simulink model "penduloInvNoLinealRealimentado"  (Simulink 7.9)
settings: Solver=ode45  StartTime=0.0  StopTime=60  RelTol=1e-3
values from neighbouring files (symbols this model uses):
  K = lqr(A,B,Q,R)    [LQR.m]    (also in bestQ.m = setK_lqr(Q_i); graficosPenduloReal.m = setK_lqr(Q_optimo))
libraries: simulink x5
settings Model: Creator=root  LastModifiedBy=root
settings SFSimCC: SimParseCustomCode=off
settings GRTTargetCC: CombineOutputUpdateFcns=off  GRTInterface=on

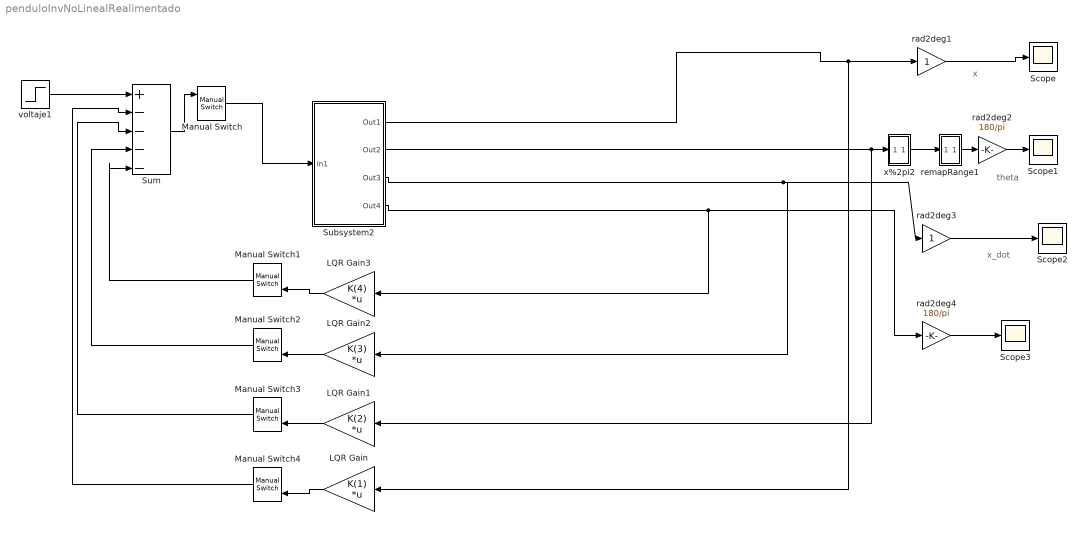
== system penduloInvNoLinealRealimentado ==
  note: x
  note: theta
  note: x_dot
  LQR Gain : Gain  Gain=K(1)  Multiplication=Matrix(K*u)  SaturateOnIntegerOverflow=on  OutDataTypeStr=Inherit: Same as input  ParamDataTypeStr=Inherit: Same as input
  LQR Gain1 : Gain  Gain=K(2)  Multiplication=Matrix(K*u)  SaturateOnIntegerOverflow=on  OutDataTypeStr=Inherit: Same as input  ParamDataTypeStr=Inherit: Same as input
  LQR Gain2 : Gain  Gain=K(3)  Multiplication=Matrix(K*u)  SaturateOnIntegerOverflow=on  OutDataTypeStr=Inherit: Same as input  ParamDataTypeStr=Inherit: Same as input
  LQR Gain3 : Gain  Gain=K(4)  Multiplication=Matrix(K*u)  SaturateOnIntegerOverflow=on  OutDataTypeStr=Inherit: Same as input  ParamDataTypeStr=Inherit: Same as input
  Manual Switch : simulink/Signal Routing/Manual Switch  sw=1  action=0  varsize=off
  Manual Switch{1..4} (4 alike) : simulink/Signal Routing/Manual Switch  sw=0  action=0  varsize=off
  Scope{,1..3} (4 alike) : Scope
      Scope settings: SaveName=ScopeData6
      Scope1 settings: SaveName=ScopeData7
      Scope2 settings: SaveName=ScopeData8
      Scope3 settings: SaveName=ScopeData9
  Subsystem2 : Subsystem
  Sum : Sum  Inputs=|+----
  rad2deg1 : Gain  SaturateOnIntegerOverflow=on  OutDataTypeStr=Inherit: Same as input  ParamDataTypeStr=Inherit: Same as input
  rad2deg2 : Gain  Gain=180/pi  SaturateOnIntegerOverflow=on  OutDataTypeStr=Inherit: Same as input  ParamDataTypeStr=Inherit: Same as input
  rad2deg3 : Gain  SaturateOnIntegerOverflow=on  OutDataTypeStr=Inherit: Same as input  ParamDataTypeStr=Inherit: Same as input
  rad2deg4 : Gain  Gain=180/pi  SaturateOnIntegerOverflow=on  OutDataTypeStr=Inherit: Same as input  ParamDataTypeStr=Inherit: Same as input
  remapRange1 : MATLAB Function  TreatAsAtomicUnit=on
  voltaje1 : Step  Time=0  After=0  SampleTime=0
  x%2pi2 : MATLAB Function  TreatAsAtomicUnit=on
  wires:
  rad2deg4/1 -> Scope3/1
  rad2deg3/1 -> Scope2/1
  Subsystem2/3(Out3) -> LQR Gain2/1, rad2deg3/1
  rad2deg1/1 -> Scope/1
  Subsystem2/1(Out1) -> rad2deg1/1, LQR Gain/1
  Subsystem2/2(Out2) -> LQR Gain1/1, x%2pi2/1(u)
  x%2pi2/1(y) -> remapRange1/1(value)
  LQR Gain3/1 -> Manual Switch1/2
  LQR Gain2/1 -> Manual Switch2/2
  LQR Gain1/1 -> Manual Switch3/2
  LQR Gain/1 -> Manual Switch4/2
  Manual Switch/1 -> Subsystem2/1(In1)
  Subsystem2/4(Out4) -> rad2deg4/1, LQR Gain3/1
  voltaje1/1 -> Sum/1
  Sum/1 -> Manual Switch/1
  Manual Switch1/1 -> Sum/5
  Manual Switch2/1 -> Sum/4
  Manual Switch3/1 -> Sum/3
  Manual Switch4/1 -> Sum/2
  remapRange1/1(y) -> rad2deg2/1
  rad2deg2/1 -> Scope1/1

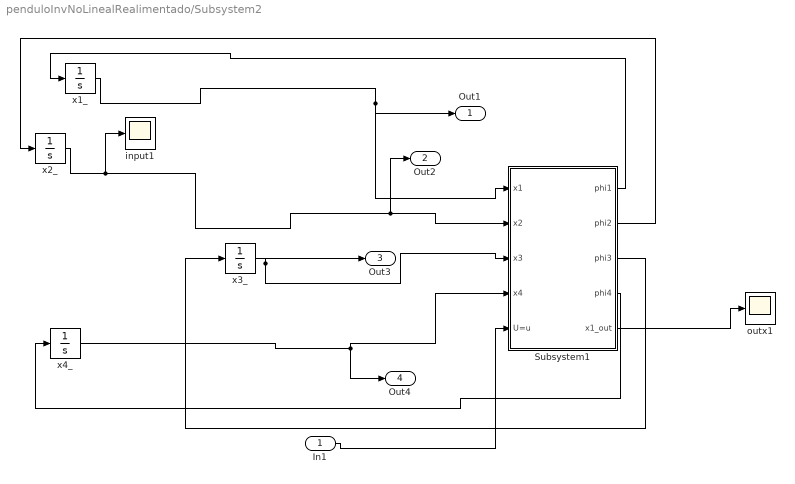
== system penduloInvNoLinealRealimentado/Subsystem2 ==
  In1 : Inport
  Subsystem1 : Subsystem
  input1 : Scope
      settings: SaveName=ScopeData5
  outx1 : Scope
  x1_ : Integrator  LimitOutput=on  UpperSaturationLimit=50  LowerSaturationLimit=-50
  x2_ : Integrator  InitialCondition=170*pi/180  UpperSaturationLimit=2*pi  LowerSaturationLimit=0
  x3_ : Integrator  LimitOutput=on  UpperSaturationLimit=0.5  LowerSaturationLimit=-0.5
  x4_ : Integrator  LimitOutput=on  UpperSaturationLimit=0.5  LowerSaturationLimit=-0.5
  Out1 : Outport
  Out2 : Outport  Port=2
  Out3 : Outport  Port=3
  Out4 : Outport  Port=4
  wires:
  x1_/1 -> Out1/1, Subsystem1/1(x1)
  Subsystem1/1(phi1) -> x1_/1
  Subsystem1/2(phi2) -> x2_/1
  Subsystem1/3(phi3) -> x3_/1
  Subsystem1/4(phi4) -> x4_/1
  x4_/1 -> Out4/1, Subsystem1/4(x4)
  x2_/1 -> input1/1, Out2/1, Subsystem1/2(x2)
  Subsystem1/5(x1_out) -> outx1/1
  In1/1 -> Subsystem1/5(U=u)
  x3_/1 -> Out3/1, Subsystem1/3(x3)

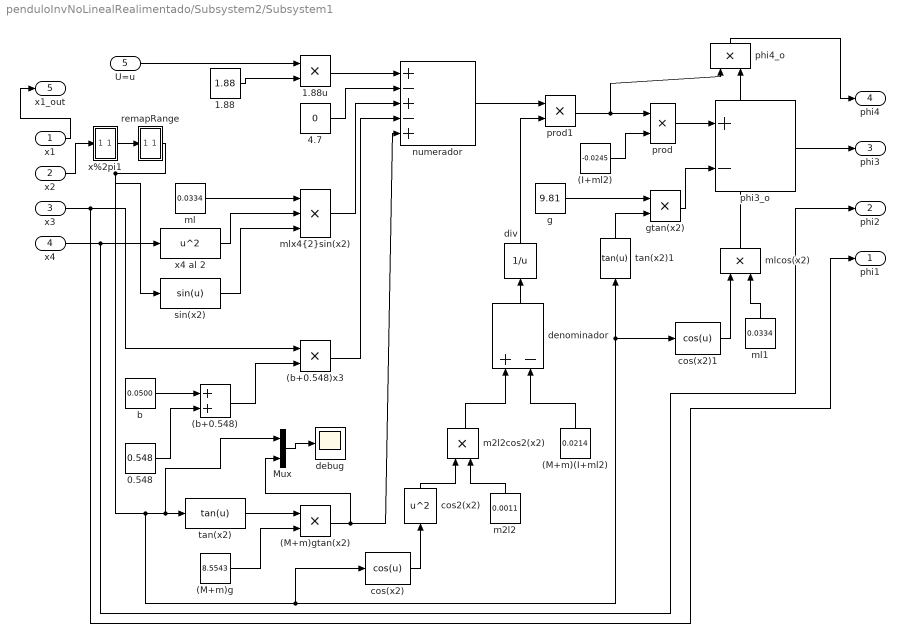
== system penduloInvNoLinealRealimentado/Subsystem2/Subsystem1 ==
  x1 : Inport
  x2 : Inport  Port=2
  x3 : Inport  Port=3
  x4 : Inport  Port=4
  U=u : Inport  Port=5
  (I+ml2) : Constant  Value=-0.0245
  (M+m)(I+ml2) : Constant  Value=0.0214
  (M+m)g : Constant  Value=8.5543
  (M+m)gtan(x2) : Product  RndMeth=Zero
  (b+0.548) : Sum
  (b+0.548)x3 : Product  RndMeth=Zero
  0.548 : Constant  Value=0.548
  1.88 : Constant  Value=1.88
  1.88u : Product  RndMeth=Zero
  4.7 : Constant  Value=0
  Mux : Mux  Inputs=2
  b : Constant  Value=0.0500
  cos(x2) : Fcn  Expr=cos(u)  SampleTime=0.1
  cos(x2)1 : Fcn  Expr=cos(u)  SampleTime=0.1
  cos2(x2) : Fcn  Expr=u^2  SampleTime=0.1
  debug : Scope
      settings: SaveName=debug
  denominador : Sum  Inputs=+-
  div : Fcn  Expr=1/u  SampleTime=0.1
  g : Constant  Value=9.81
  gtan(x2) : Product  RndMeth=Zero
  m2l2 : Constant  Value=0.0011
  m2l2cos2(x2) : Product  RndMeth=Zero
  ml : Constant  Value=0.0334
  ml1 : Constant  Value=0.0334
  mlcos(x2) : Product  RndMeth=Zero
  "mlx4{2}sin(x2)" : Product  Inputs=3  RndMeth=Zero
  numerador : Sum  Inputs=+-+-+
  phi3_o : Sum  Inputs=+-
  phi4_o : Product  RndMeth=Zero
  prod : Product  RndMeth=Zero
  prod1 : Product  RndMeth=Zero
  remapRange : MATLAB Function  TreatAsAtomicUnit=on
  sin(x2) : Fcn  Expr=sin(u)  SampleTime=0.1
  tan(x2) : Fcn  Expr=tan(u)  SampleTime=0.1
  tan(x2)1 : Fcn  Expr=tan(u)  SampleTime=0.1
  x%2pi1 : MATLAB Function  TreatAsAtomicUnit=on
  x4 al 2 : Fcn  Expr=u^2  SampleTime=0.1
  phi1 : Outport
  phi2 : Outport  Port=2
  phi3 : Outport  Port=3
  phi4 : Outport  Port=4
  x1_out : Outport  Port=5
  wires:
  1.88/1 -> 1.88u/2
  U=u/1 -> 1.88u/1
  1.88u/1 -> numerador/1
  4.7/1 -> numerador/2
  ml/1 -> "mlx4{2}sin(x2)"/1
  sin(x2)/1 -> "mlx4{2}sin(x2)"/3
  x4 al 2/1 -> "mlx4{2}sin(x2)"/2
  x4/1 -> x4 al 2/1, phi2/1
  "mlx4{2}sin(x2)"/1 -> numerador/3
  (b+0.548)x3/1 -> numerador/4
  x3/1 -> phi1/1, (b+0.548)x3/1
  (b+0.548)/1 -> (b+0.548)x3/2
  b/1 -> (b+0.548)/1
  0.548/1 -> (b+0.548)/2
  (M+m)gtan(x2)/1 -> numerador/5, Mux/2
  tan(x2)/1 -> (M+m)gtan(x2)/1
  (M+m)g/1 -> (M+m)gtan(x2)/2
  (M+m)(I+ml2)/1 -> denominador/2
  m2l2cos2(x2)/1 -> denominador/1
  cos2(x2)/1 -> m2l2cos2(x2)/1
  m2l2/1 -> m2l2cos2(x2)/2
  cos(x2)/1 -> cos2(x2)/1
  numerador/1 -> prod1/1
  prod1/1 -> prod/1, phi4_o/1
  (I+ml2)/1 -> prod/2
  prod/1 -> phi3_o/1
  gtan(x2)/1 -> phi3_o/2
  g/1 -> gtan(x2)/1
  tan(x2)1/1 -> gtan(x2)/2
  mlcos(x2)/1 -> phi4_o/2
  ml1/1 -> mlcos(x2)/2
  cos(x2)1/1 -> mlcos(x2)/1
  phi3_o/1 -> phi3/1
  phi4_o/1 -> phi4/1
  denominador/1 -> div/1
  div/1 -> prod1/2
  x1/1 -> x1_out/1
  Mux/1 -> debug/1
  x%2pi1/1(y) -> remapRange/1(value)
  remapRange/1(y) -> cos(x2)/1, tan(x2)1/1, cos(x2)1/1, tan(x2)/1, Mux/1, sin(x2)/1
  x2/1 -> x%2pi1/1(u)

== matlab function Subsystem2/Subsystem1/remapRange ==
  data: value input double; y output double
function y = remapRange(value)
    scaleFactor = pi/180;
    if (value>180*scaleFactor)
        %constants
        fromLow = 181*scaleFactor;
        fromHigh = 360*scaleFactor;
        toLow = -179*scaleFactor;
        toHigh = 0*scaleFactor;
        %calculations
        new_range = toHigh-toLow;
        old_range = fromHigh - fromLow;
        new_value = (new_range/old_range)*(value-fromLow)+toLow;
        y = new_value;
    else
        y = value;
    end
        
end

== matlab function Subsystem2/Subsystem1/x%2pi1 ==
  data: u input double; y output double
function y = fcn(u)
%#codegen

    y = mod(u,2*pi);
end

== matlab function remapRange1 ==
  data: value input double; y output double
function y = remapRange(value)
    scaleFactor = pi/180;
    if (value>180*scaleFactor)
        %constants
        fromLow = 181*scaleFactor;
        fromHigh = 360*scaleFactor;
        toLow = -179*scaleFactor;
        toHigh = 0*scaleFactor;
        %calculations
        new_range = toHigh-toLow;
        old_range = fromHigh - fromLow;
        new_value = (new_range/old_range)*(value-fromLow)+toLow;
        y = new_value;
    else
        y = value;
    end
        
end

== matlab function x%2pi2 ==
  data: u input double; y output double
function y = fcn(u)
%#codegen

    y = mod(u,2*pi);
end
